simulink model "RM3_cHydraulic_PTO_WithSimscape"  (R2020b)
settings: Solver=ode4  StartTime=0  StopTime=400  FixedStep=0.001  MaxStep=0.001  RelTol=1e-3
values from neighbouring files (symbols this model uses):
  Apiston = 0.0378    [ptoSimInputFile.m]
  Disp_max = 1.9794e+03    (= 1979.4)    [ptoSimInputFile.m]
  fric_shaftHM = 0.05    [ptoSimInputFile.m]
  J_shaftHM = 20    [ptoSimInputFile.m]
  ptosim = ptoSimClass('Compressible Fluid Hydraulic')    [ptoSimInputFile.m]
  Vo_cylinder = 15*Apiston    (= 0.567)    [ptoSimInputFile.m]
undefined symbols (not defined in the file or in its folder): body, constraint, pto
libraries: fl_lib x21, nesl_utility x12, sh_lib x8, WECSim_Lib x5, PTOSim_Lib x1
settings Model: Creator=jleonqu  LastModifiedBy=jleonqu
settings SolverCC: ZeroCrossControl=DisableAll  AutoInsertRateTranBlk=on
settings DataIOCC: ReturnWorkspaceOutputs=off
settings OptimizationCC: SimCompilerOptimization=on

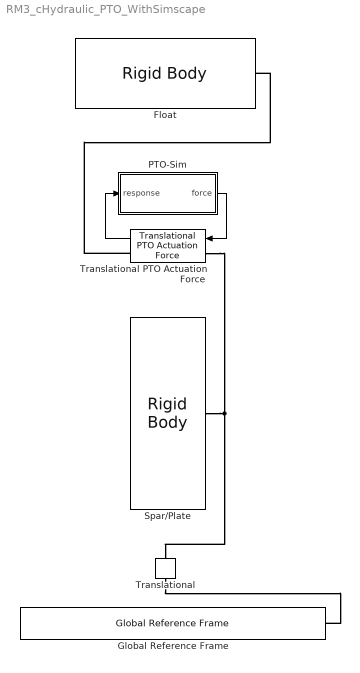
== system RM3_cHydraulic_PTO_WithSimscape ==
  Float : WECSim_Lib/Body Elements/Rigid Body  body=body(1)
      settings: AttributesFormatString=%<body>  SourceProductName=WEC-Sim
  Global Reference Frame : WECSim_Lib/Frames/Global Reference Frame  waves=waves  simu=simu
      settings: SourceProductName=WEC-Sim
  PTO-Sim : Subsystem
  Spar/Plate : WECSim_Lib/Body Elements/Rigid Body  body=body(2)
      settings: AttributesFormatString=%<body>  SourceProductName=WEC-Sim
  Translational : WECSim_Lib/Constraints/Translational  constraint=constraint(1)
      settings: AttributesFormatString=%<constraint>  SourceProductName=WEC-Sim
  Translational PTO Actuation Force : WECSim_Lib/PTOs/Translational PTO Actuation Force  pto=pto(1)
      settings: AttributesFormatString=%<pto>  SourceProductName=WEC-Sim
  wires:
  PTO-Sim/1(force) -> Translational PTO Actuation Force/1
  Translational PTO Actuation Force/1 -> PTO-Sim/1(response)
  connections:
  Translational PTO Actuation Force/LConn1 -- Spar/Plate/RConn1 -- Translational/RConn1
  Translational/LConn1 -- Global Reference Frame/RConn1
  Translational PTO Actuation Force/RConn1 -- Float/RConn1

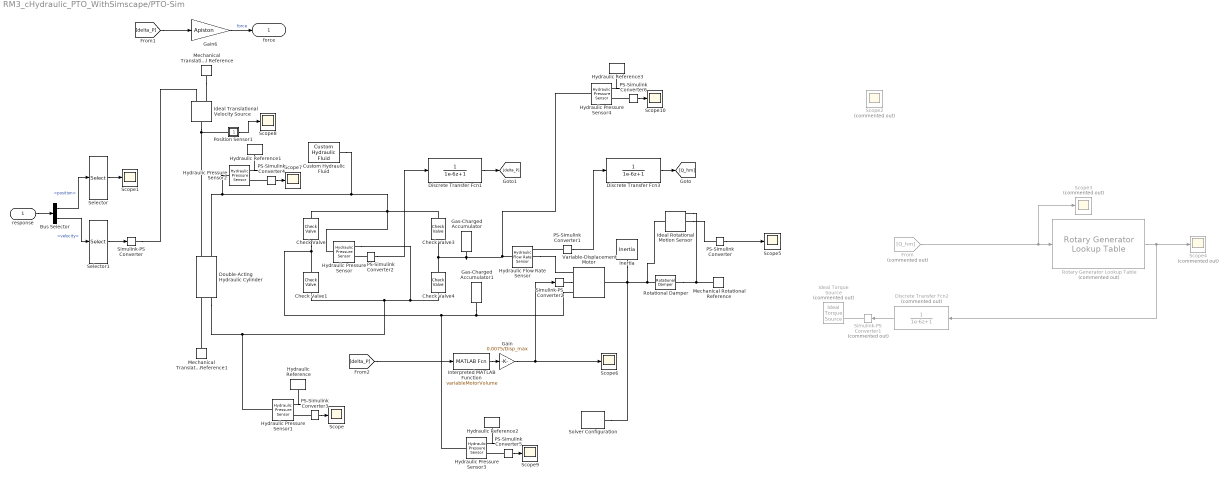
== system RM3_cHydraulic_PTO_WithSimscape/PTO-Sim ==
  response : Inport
  Bus Selector : BusSelector  OutputSignals=position,velocity
  Check Valve{,1,3..4} (4 alike) : sh_lib/Valves/Directional Valves/Check Valve  area_max=Amax_Check m^2  pres_crack=pMin_Check Pa  pres_max=pMax_Check Pa  C_d=Cd_Check  A_leak=1e-12 m^2  lam_spec=1  B_lam=0.999  Re_cr=12  dynamic=0  tau=0.1 s  area_init=1e-12 m^2
      settings: SourceProductBaseCode=SH  InternalSimscapePortConfiguration="{\"Bottom\":[],\"Left\":[{\"id\":\"A\",\"label\":\"A\",\"type\":\"foundation.hydraulic.hydraulic\"}],\"Right\":[{\"id\":\"B\",\"label\":\"B\",\"type\":\"foundation.hydraulic.hydraulic\"}],\"Top\":[]}"
  Custom Hydraulic Fluid : fl_lib/Hydraulic/Hydraulic Utilities/Custom Hydraulic Fluid  density=850 kg/m^3  viscosity_kin=18e-6 m^2/s  bulk=1.86e9 Pa  alpha=0.005  range_error=2
      settings: SourceProductBaseCode=SS  InternalSimscapePortConfiguration="{\"Bottom\":[],\"Left\":[],\"Right\":[{\"id\":\"G\",\"label\":\"\",\"type\":\"foundation.hydraulic.hydraulic\"}],\"Top\":[]}"
  Discrete Transfer Fcn1 : DiscreteTransferFcn  Denominator=[1e-6 1]
  Discrete Transfer Fcn2 : DiscreteTransferFcn  Commented=on  Denominator=[1e-6 1]
  Discrete Transfer Fcn3 : DiscreteTransferFcn  Denominator=[1e-6 1]
  Double-Acting Hydraulic Cylinder : sh_lib/Hydraulic Cylinders/Double-Acting Hydraulic Cylinder  area_A=Apiston m^2  area_B=Apiston m^2  stroke=2*Vo_cylinder/Apiston m  init_pos=0.3*2*Vo_cylinder/Apiston m  dead_vol_A=1e-4 m^3  dead_vol_B=1e-4 m^3  init_pressure_A=0 Pa  init_pressure_B=0 Pa  k_sh=1.4  stiff=1e6 N/m  D=150 N/(m/s)  hardstop_model=1  transition=0.1 mm  or=1
      settings: SourceProductBaseCode=SH  InternalSimscapePortConfiguration="{\"Bottom\":[],\"Left\":[{\"id\":\"C\",\"label\":\"C\",\"type\":\"foundation.mechanical.translational.translational\"},{\"id\":\"A\",\"label\":\"A\",\"type\":\"foundation.hydraulic.hydraulic\"}],\"Right\":[{\"id\":\"R\",\"label\":\"R\",\"type\":\"foundation.mechanical.translational.translational\"},{\"id\":\"B\",\"label\":\"B\",\"type\":\"foundation.hydraulic.hydraulic\"}],\"Top\":[]}"
  From : From  Commented=on  GotoTag=Q_hm
  Gain : Gain  Gain=0.0075/Disp_max
  Gain6 : Gain  Gain=Apiston
  Gas-Charged Accumulator : sh_lib/Accumulators/Gas-Charged Accumulator  capacity=VI0_HPAcc m^3  dead_volume=4e-5 m^3  pr_preload=pIprecharge_HPAcc Pa  k_sh=1.4  stiff_coeff=1e10 Pa/m^3  penetr_coeff=1e10 s*Pa/m^6  flow_rate_specify=off  flow_rate_priority=None  flow_rate=0.005 m^3/s  flow_rate_nominal_specify=off  flow_rate_nominal_unit=m^3/s  flow_rate_nominal_value=1  liquid_volume_specify=off  liquid_volume_priority=High  liquid_volume=0.005 m^3  liquid_volume_nominal_specify=off  liquid_volume_nominal_unit=m^3  liquid_volume_nominal_value=1  liquid_pressure_specify=off  liquid_pressure_priority=None  liquid_pressure=1.01325e+5 Pa  liquid_pressure_nominal_specify=off  liquid_pressure_nominal_unit=Pa  liquid_pressure_nominal_value=1
      settings: SourceProductBaseCode=SH  InternalSimscapePortConfiguration="{\"Bottom\":[],\"Left\":[],\"Right\":[{\"id\":\"A\",\"label\":\"A\",\"type\":\"foundation.hydraulic.hydraulic\"}],\"Top\":[]}"
  Gas-Charged Accumulator1 : sh_lib/Accumulators/Gas-Charged Accumulator  capacity=VI0_LPAcc m^3  dead_volume=4e-5 m^3  pr_preload=pIprecharge_LPAcc Pa  k_sh=1.4  stiff_coeff=1e10 Pa/m^3  penetr_coeff=1e10 s*Pa/m^6  flow_rate_specify=off  flow_rate_priority=None  flow_rate=0.005 m^3/s  flow_rate_nominal_specify=off  flow_rate_nominal_unit=m^3/s  flow_rate_nominal_value=1  liquid_volume_specify=off  liquid_volume_priority=High  liquid_volume=0.005 m^3  liquid_volume_nominal_specify=off  liquid_volume_nominal_unit=m^3  liquid_volume_nominal_value=1  liquid_pressure_specify=off  liquid_pressure_priority=None  liquid_pressure=1.01325e+5 Pa  liquid_pressure_nominal_specify=off  liquid_pressure_nominal_unit=Pa  liquid_pressure_nominal_value=1
      settings: SourceProductBaseCode=SH  InternalSimscapePortConfiguration="{\"Bottom\":[],\"Left\":[],\"Right\":[{\"id\":\"A\",\"label\":\"A\",\"type\":\"foundation.hydraulic.hydraulic\"}],\"Top\":[]}"
  Hydraulic Flow Rate Sensor : fl_lib/Hydraulic/Hydraulic Sensors/Hydraulic Flow Rate Sensor
  Hydraulic Pressure Sensor{,1..4} (5 alike) : fl_lib/Hydraulic/Hydraulic Sensors/Hydraulic Pressure Sensor
  Hydraulic Reference{,1..3} (4 alike) : fl_lib/Hydraulic/Hydraulic Elements/Hydraulic Reference
  Ideal Rotational Motion Sensor : fl_lib/Mechanical/Mechanical Sensors/Ideal Rotational Motion Sensor  wrap_angle=simscape.enum.onoff.off  offset=0 rad
  Ideal Torque Source : fl_lib/Mechanical/Mechanical Sources/Ideal Torque Source  Commented=on
  Ideal Translational Velocity Source : fl_lib/Mechanical/Mechanical Sources/Ideal Translational Velocity Source
  Inertia : fl_lib/Mechanical/Rotational Elements/Inertia  inertia=J_shaftHM*1000 kg*m^2  num_ports=foundation.enum.numPorts2.one  w_specify=off  w_priority=High  w=0 rad/s  w_nominal_specify=off  w_nominal_unit=rad/s  w_nominal_value=1  t_specify=off  t_priority=None  t=0 N*m  t_nominal_specify=off  t_nominal_unit=N*m  t_nominal_value=1
  Interpreted MATLAB Function : MATLABFcn  MATLABFcn=variableMotorVolume
  Mechanical Rotational Reference : fl_lib/Mechanical/Rotational Elements/Mechanical Rotational Reference
  Mechanical Translational Reference : fl_lib/Mechanical/Translational Elements/Mechanical Translational Reference
  Mechanical Translational Reference1 : fl_lib/Mechanical/Translational Elements/Mechanical Translational Reference
  PS-Simulink Converter{,1..6} (7 alike) : nesl_utility/PS-Simulink Converter  PhysicalDomain=network_engine_domain  SubClassName=ps_output  LeftPortType=input  RightPortType=output  PseudoPeriodic=off  Frequencies=[]  Unit=inherit  AffineConversion=off
  Position Sensor1 : Subsystem
      mask Display: disp('P');
  Rotary Generator Lookup Table : PTOSim_Lib/Generator/Rotary Generator Lookup Table  Commented=on  ptosim=ptosim.rotaryGenerator(1)
      settings: SourceProductName=PTO-Sim
  Rotational Damper : fl_lib/Mechanical/Rotational Elements/Rotational Damper  D=fric_shaftHM N*m/(rad/s)  w_specify=off  w_priority=None  w=0 rad/s  w_nominal_specify=off  w_nominal_unit=rad/s  w_nominal_value=1  t_specify=off  t_priority=None  t=0 N*m  t_nominal_specify=off  t_nominal_unit=N*m  t_nominal_value=1
  Scope{,1,5..10} (8 alike) : Scope
  Scope2 : Scope  Commented=on
  Scope3 : Scope  Commented=on
  Scope4 : Scope  Commented=on
  Selector : Selector  InputPortWidth=6  IndexOptions=Index vector (dialog)  Indices=3  OutputSizes=1
  Selector1 : Selector  InputPortWidth=6  IndexOptions=Index vector (dialog)  Indices=3  OutputSizes=1
  Simulink-PS Converter : nesl_utility/Simulink-PS Converter  PhysicalDomain=network_engine_domain  SubClassName=ps_input  LeftPortType=input  RightPortType=output  PseudoPeriodic=off  Frequencies=[]  NoiseDistribution=none  NoiseParameters=[]  Unit=1  AffineConversion=off  FilteringAndDerivatives=provide  SimscapeFilterOrder=1  InputFilterTimeConstant=0.001  UdotUserProvided=0
  Simulink-PS Converter1 : nesl_utility/Simulink-PS Converter  Commented=on  PhysicalDomain=network_engine_domain  SubClassName=ps_input  LeftPortType=input  RightPortType=output  PseudoPeriodic=off  Frequencies=[]  NoiseDistribution=none  NoiseParameters=[]  Unit=1  AffineConversion=off  FilteringAndDerivatives=provide  SimscapeFilterOrder=1  InputFilterTimeConstant=0.001  UdotUserProvided=0
  Simulink-PS Converter2 : nesl_utility/Simulink-PS Converter  PhysicalDomain=network_engine_domain  SubClassName=ps_input  LeftPortType=input  RightPortType=output  PseudoPeriodic=off  Frequencies=[]  NoiseDistribution=none  NoiseParameters=[]  Unit=1  AffineConversion=off  FilteringAndDerivatives=provide  SimscapeFilterOrder=1  InputFilterTimeConstant=0.001  UdotUserProvided=0
  Solver Configuration : nesl_utility/Solver Configuration  PhysicalDomain=network_engine_domain  SubClassName=solver  LeftPortType=input  RightPortType=generic  Tones=[]  Harmonics=[]  SimulateNoise=off  Profile=off  UseLocalSampling=off  EnableSwitchedLinearOptims=on  FrequencyDomain=off  UseCCode=off  RelTol=0.001  AbsTol=1e-06  MinStep=1e-09  ToWorkspace=off  RevertToSquareIcSolve=off  NumHomotopyIterations=100  PhasorMode=off  PhasorModeNumHarmonics=1  DoDC=off  ResidualTolerance=1e-09  UseLocalSolver=on  LocalSolverChoice=NE_BACKWARD_EULER_ADVANCER  LocalSolverSampleTime=0.001  DoFixedCost=on  MaxNonlinIter=5  MaxModeIter=2  ComputeImpulses=off  ImpulseIterations=2  LinearAlgebra=Full  EquationFormulation=NE_TIME_EF  DelaysMemoryBudget=1024  AutomaticFiltering=on  FilteringTimeConstant=0.001  PartitionStorageMethod=AS_NEEDED  PartitionMemoryBudget=1024  PartitionMethod=ROBUST
  Variable-Displacement Motor : sh_lib/Pumps and Motors/Variable-Displacement Motor  mdl_type=2  stroke_max=0.005 m  D_max=Disp_max cm^3/rev  cntrl_mem_tab=[-.0075, 0, .0075] m  displ_tab=[Disp_max, 0, Disp_max] cm^3/rev  interp_method=1  extrap_method=1  loss_spec=1  w_nominal=188 rad/s  pr_nominal=100e5 Pa  visc_nominal=18 cSt  dens_nominal=900 kg/m^3  efficiency_vol=0.92  no_load_torque=0.05 N*m  torque_pressure_coeff=0.6e-6 N*m/Pa  p_diff_eff_TLU=[100000, 1000000, 2000000] Pa  omega_eff_TLU=[25, 50, 100, 200, 300, 400] rad/s  displacement_eff_TLU=[-30, -19, 19, 30] cm^3/rev  vol_eff_TLU=repmat([.816, .908, .954, .977, .981, .984; .325, .663, .831, .916, .925, .946; .137, .568, .78, .892, .893, .91], 1, 1, 4)  mech_eff_TLU=repmat([.996, .996, .996, .996, .996, .996; .988, .989, .989, .989, .989, .99; .981, .981, .982, .982, .983, .984], 1, 1, 4)  p_diff_loss_TLU=[100000, 1000000, 2000000] Pa  omega_loss_TLU=[25, 50, 100, 200, 300, 400] rad/s  displacement_loss_TLU=[-30, -19, 19, 30] cm^3/rev  vol_loss_TLU=repmat([.0282, .0253, .0241, .0235, .0291, .0325; .2596, .1271, .1017, .0917, .1216, .1142; .7874, .1901, .141, .1211, .1797, .1978] * 1e-3, 1, 1, 4) m^3/s  mech_loss_TLU=repmat([.002, .002, .002, .002, .002, .002; .06, .055, .055, .055, .055, .05; .19, .19, .18, .18, .17, .16], 1, 1, 4) N*m  pressure_threshold=1e5 Pa  omega_threshold=10 rad/s  displacement_threshold=0.5 cm^3/rev  octant_check=0  pressure_check=0  min_valid_pressure=0 Pa  vol_eff_min=1e-3  vol_eff_max=1  mech_eff_min=1e-3  mech_eff_max=1
      settings: SourceProductBaseCode=SH  InternalSimscapePortConfiguration="{\"Bottom\":[],\"Left\":[{\"id\":\"A\",\"label\":\"A\",\"type\":\"foundation.hydraulic.hydraulic\"},{\"id\":\"C\",\"label\":\"C\",\"type\":\"input\"},{\"id\":\"B\",\"label\":\"B\",\"type\":\"foundation.hydraulic.hydraulic\"}],\"Right\":[{\"id\":\"S\",\"label\":\"S\",\"type\":\"foundation.mechanical.rotational.rotational\"}],\"Top\":[]}"
  force : Outport  VectorParamsAs1DForOutWhenUnconnected=off
  wires:
  response/1 -> Bus Selector/1
  Bus Selector/1 -> Selector/1  "<position>"
  Bus Selector/2 -> Selector1/1  "<velocity>"
  Selector1/1 -> Simulink-PS Converter/1
  Position Sensor1/1(P) -> Scope8/1
  PS-Simulink Converter1/1 -> Discrete Transfer Fcn3/1
  From/1 -> Scope3/1, Rotary Generator Lookup Table/2
  PS-Simulink Converter2/1 -> Discrete Transfer Fcn1/1
  [delta_P] -> Gain6/1
  Gain6/1 -> force/1  "force"
  Selector/1 -> Scope1/1
  PS-Simulink Converter/1 -> Scope5/1
  Interpreted MATLAB Function/1 -> Gain/1
  Gain/1 -> Scope6/1, Simulink-PS Converter2/1
  Rotary Generator Lookup Table/1 -> Discrete Transfer Fcn2/1, Scope4/1
  Discrete Transfer Fcn2/1 -> Simulink-PS Converter1/1
  Discrete Transfer Fcn1/1 -> [delta_P]
  [delta_P] -> Interpreted MATLAB Function/1
  Discrete Transfer Fcn3/1 -> [Q_hm]
  PS-Simulink Converter3/1 -> Scope/1
  PS-Simulink Converter4/1 -> Scope7/1
  PS-Simulink Converter5/1 -> Scope9/1
  PS-Simulink Converter6/1 -> Scope10/1
  connections:
  Mechanical Translational Reference1/LConn1 -- Double-Acting Hydraulic Cylinder/LConn1
  Ideal Translational Velocity Source/LConn1 -- Position Sensor1/LConn1 -- Double-Acting Hydraulic Cylinder/RConn1
  Mechanical Translational Reference/LConn1 -- Ideal Translational Velocity Source/RConn2
  Simulink-PS Converter/RConn1 -- Ideal Translational Velocity Source/RConn1
  Check Valve/LConn1 -- Hydraulic Pressure Sensor3/LConn1 -- Variable-Displacement Motor/LConn3 -- Gas-Charged Accumulator1/RConn1 -- Check Valve1/LConn1
  Hydraulic Pressure Sensor4/LConn1 -- Hydraulic Flow Rate Sensor/LConn1 -- Gas-Charged Accumulator/RConn1 -- Check Valve4/RConn1 -- Check Valve3/RConn1
  Check Valve/RConn1 -- Hydraulic Pressure Sensor2/LConn1 -- Double-Acting Hydraulic Cylinder/RConn2 -- Custom Hydraulic Fluid/RConn1 -- Check Valve3/LConn1 -- Hydraulic Pressure Sensor/LConn1
  Double-Acting Hydraulic Cylinder/LConn2 -- Hydraulic Pressure Sensor1/LConn1 -- Check Valve1/RConn1 -- Check Valve4/LConn1 -- Hydraulic Pressure Sensor/RConn1
  Ideal Rotational Motion Sensor/RConn2 -- PS-Simulink Converter/LConn1
  Hydraulic Flow Rate Sensor/RConn2 -- Variable-Displacement Motor/LConn1
  PS-Simulink Converter1/LConn1 -- Hydraulic Flow Rate Sensor/RConn1
  PS-Simulink Converter2/LConn1 -- Hydraulic Pressure Sensor/RConn2
  Rotational Damper/LConn1 -- Ideal Rotational Motion Sensor/LConn1 -- Solver Configuration/RConn1 -- Inertia/LConn1 -- Variable-Displacement Motor/RConn1
  Rotational Damper/RConn1 -- Ideal Rotational Motion Sensor/RConn1 -- Mechanical Rotational Reference/LConn1
  Simulink-PS Converter1/RConn1 -- Ideal Torque Source/RConn1
  Simulink-PS Converter2/RConn1 -- Variable-Displacement Motor/LConn2
  Hydraulic Pressure Sensor1/RConn1 -- Hydraulic Reference/LConn1
  PS-Simulink Converter3/LConn1 -- Hydraulic Pressure Sensor1/RConn2
  Hydraulic Pressure Sensor2/RConn1 -- Hydraulic Reference1/LConn1
  PS-Simulink Converter4/LConn1 -- Hydraulic Pressure Sensor2/RConn2
  Hydraulic Pressure Sensor3/RConn1 -- Hydraulic Reference2/LConn1
  PS-Simulink Converter5/LConn1 -- Hydraulic Pressure Sensor3/RConn2
  Hydraulic Pressure Sensor4/RConn1 -- Hydraulic Reference3/LConn1
  PS-Simulink Converter6/LConn1 -- Hydraulic Pressure Sensor4/RConn2

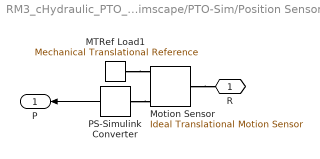
== system RM3_cHydraulic_PTO_WithSimscape/PTO-Sim/Position Sensor1 ==
  MTRef Load1 : fl_lib/Mechanical/Translational Elements/Mechanical Translational Reference  Tag=Factory Generic
  Motion Sensor : fl_lib/Mechanical/Mechanical Sensors/Ideal Translational Motion Sensor  offset=0 m
  PS-Simulink Converter : nesl_utility/PS-Simulink Converter  PhysicalDomain=network_engine_domain  SubClassName=ps_output  LeftPortType=input  RightPortType=output  PseudoPeriodic=off  Frequencies=[]  Unit=1  AffineConversion=off
  R : PMIOPort  Side=Left
  P : Outport  VectorParamsAs1DForOutWhenUnconnected=off
  wires:
  PS-Simulink Converter/1 -> P/1
  connections:
  PS-Simulink Converter/LConn1 -- Motion Sensor/RConn3
  Motion Sensor/LConn1 -- R/RConn1
  MTRef Load1/LConn1 -- Motion Sensor/RConn1
